simulink model "Week3_Sum2"  (R2020b)
settings: Solver=VariableStepAuto  StartTime=0.0  StopTime=10.0  RelTol=1e-3
undefined symbols (not defined in the file or in its folder): DiscIntNeverNeededParam
libraries: simulink x1
settings Model: Creator=Aradhana desai  LastModifiedBy=Aradhana desai

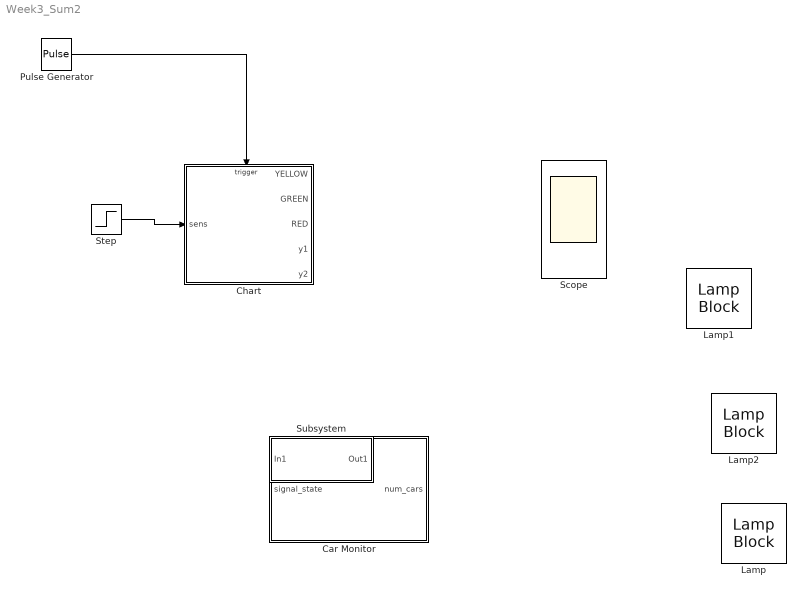
== system Week3_Sum2 ==
  Car Monitor : Subsystem
  Chart : Stateflow chart  TreatAsAtomicUnit=on
  Lamp : LampBlock
  Lamp1 : LampBlock
  Lamp2 : LampBlock
  Pulse Generator : DiscretePulseGenerator  PulseType=Time based  Period=0.04  PulseWidth=50
  Scope : Scope  NumInputPorts=5
  Step : Step  SampleTime=0
  Subsystem : Subsystem
  wires:
  Pulse Generator/1 -> Chart/Trigger
  ? -> Scope/4
  ? -> Scope/5
  Step/1 -> Chart/1(sens)

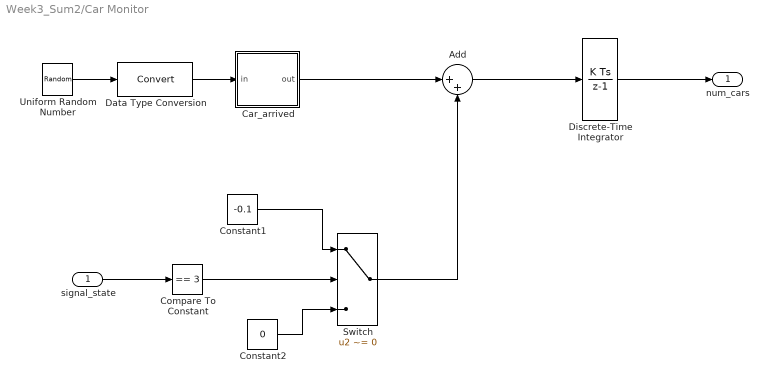
== system Week3_Sum2/Car Monitor ==
  signal_state : Inport
  Add : Sum  Inputs=|++
  Car_arrived : Stateflow chart  TreatAsAtomicUnit=on
  Compare To Constant : simulink/Logic and Bit Operations/Compare To Constant  relop===  const=3  OutDataTypeStr=boolean  ZeroCross=off
  Constant1 : Constant  Value=-0.1
  Constant2 : Constant  Value=0
  Data Type Conversion : DataTypeConversion
  Discrete-Time Integrator : DiscreteIntegrator  SampleTime=-1  LimitOutput=on  LowerSaturationLimit=0  ICPrevOutput=DiscIntNeverNeededParam  ICPrevScaledInput=DiscIntNeverNeededParam
  Switch : Switch  Criteria=u2 ~= 0
  Uniform Random Number : UniformRandomNumber  Minimum=0  Maximum=100  Seed=177836  SampleTime=0
  num_cars : Outport  VectorParamsAs1DForOutWhenUnconnected=off
  wires:
  Car_arrived/1(out) -> Add/1
  Uniform Random Number/1 -> Data Type Conversion/1
  Constant1/1 -> Switch/1
  Constant2/1 -> Switch/3
  Compare To Constant/1 -> Switch/2
  Data Type Conversion/1 -> Car_arrived/1(in)
  signal_state/1 -> Compare To Constant/1
  Discrete-Time Integrator/1 -> num_cars/1
  Switch/1 -> Add/2
  Add/1 -> Discrete-Time Integrator/1

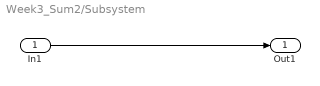
== system Week3_Sum2/Subsystem ==
  In1 : Inport
  Out1 : Outport
  wires:
  In1/1 -> Out1/1

== stateflow chart Week3_Sum2/Chart ==
  state Stop
    y1=RED;
    y2=GREEN;
  state StopForTraffic
    y1=RED;
    y2=GREEN
  state StopToGo
    y1=RED;
    y2=YELLOW;
  state GotoStop
    y1=YELLOW;
    y2=RED;
  state Go
    y1=GREEN;
    y2=RED;
  (default) -> Stop
  Stop -> StopForTraffic : after(20,tick)
  StopForTraffic -> StopToGo : [sens]
  GotoStop -> Stop : after(3,tick)
  StopToGo -> Go : after(3,tick)
  Go -> GotoStop : after(10,tick)
  data: sens input boolean; YELLOW output; GREEN output; RED output; y1 output uint8; y2 output uint8
  events: pulse input RISING_EDGE_EVENT

== stateflow chart Week3_Sum2/Car Monitor/Car_arrived ==
  (default) -> (junction 2) : {out = in > 98;}
  data: in input int8; out output double
